simulink model "Compressor"  (R2015b)
settings: Solver=FixedStepDiscrete  StartTime=0.0  StopTime=10.0  RelTol=1e-3
undefined symbols (not defined in the file or in its folder): cp_air, etaCmax, etaCmin, gamma_air, Nc, p01, pCref, PiC, PiC_at_etaCmax, PsiMax, Q11, Q12, Q22, rComp, T01, TCref, WcCorr_at_etaCmax, WcCorrMax
settings Model: Creator=fahle  LastModifiedBy=fahle

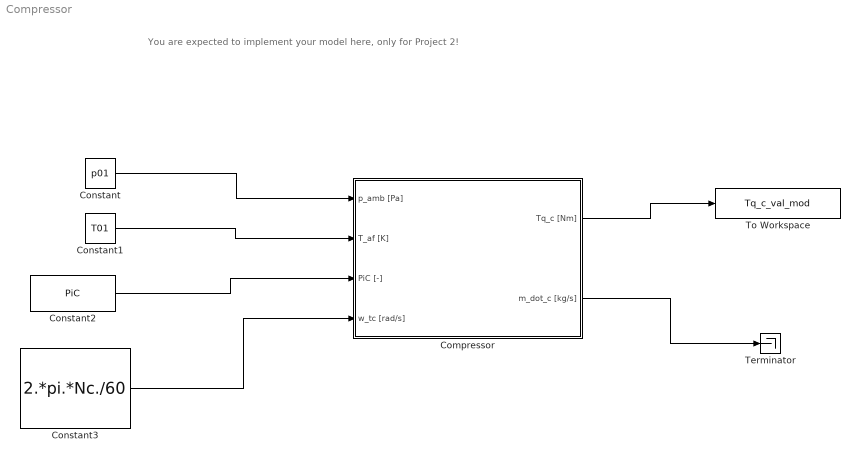
== system Compressor ==
  note: You are expected to implement your model here, only for Project 2!
  Compressor : Subsystem
  Constant : Constant  Value=p01
  Constant1 : Constant  Value=T01
  Constant2 : Constant  Value=PiC
  Constant3 : Constant  Value=2.*pi.*Nc./60
  Terminator : Terminator
  To Workspace : ToWorkspace  VariableName=Tq_c_val_mod  SampleTime=-1
      settings: Save2DSignal=2-D array (concatenate along first dimension)
  wires:
  Compressor/1(Tq_c [Nm]) -> To Workspace/1
  Compressor/2(m_dot_c [kg/s]) -> Terminator/1
  Constant3/1 -> Compressor/4(w_tc [rad/s])
  Constant2/1 -> Compressor/3(PiC [-])
  Constant1/1 -> Compressor/2(T_af [K])
  Constant/1 -> Compressor/1(p_amb [Pa])

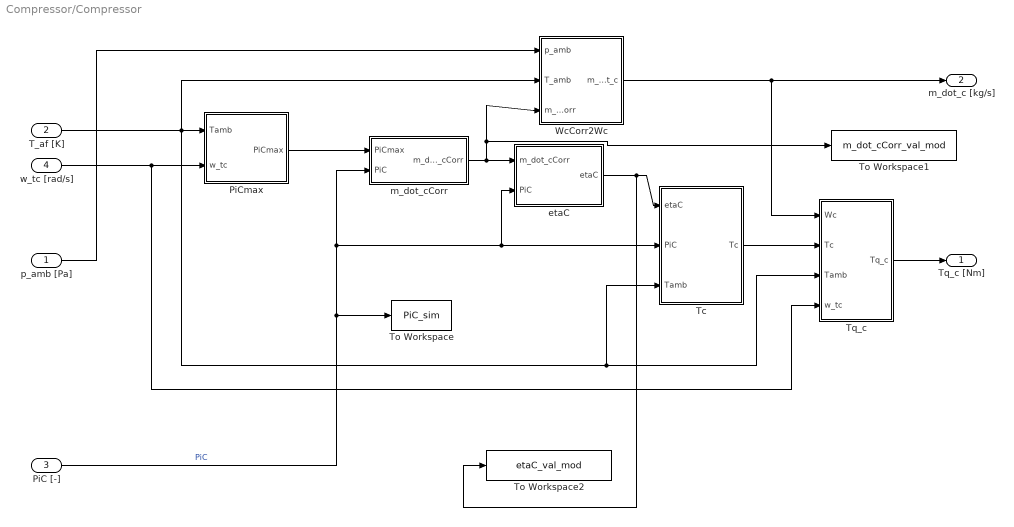
== system Compressor/Compressor ==
  p_amb [Pa] : Inport
  T_af [K] : Inport  Port=2
  PiC [-] : Inport  Port=3
  w_tc [rad/s] : Inport  Port=4
  PiCmax : Subsystem
  Tc : Subsystem
  To Workspace : ToWorkspace  VariableName=PiC_sim  SampleTime=-1
  To Workspace1 : ToWorkspace  VariableName=m_dot_cCorr_val_mod  SampleTime=-1
  To Workspace2 : ToWorkspace  VariableName=etaC_val_mod  SaveFormat=Structure With Time  SampleTime=-1
  Tq_c : Subsystem
  WcCorr2Wc : Subsystem
  etaC : Subsystem
  m_dot_cCorr : Subsystem
  Tq_c [Nm] : Outport
  m_dot_c [kg/s] : Outport  Port=2
  wires:
  T_af [K]/1 -> Tq_c/3(Tamb), Tc/3(Tamb), WcCorr2Wc/2(T_amb), PiCmax/1(Tamb)
  etaC/1(etaC) -> To Workspace2/1, Tc/1(etaC)
  p_amb [Pa]/1 -> WcCorr2Wc/1(p_amb)
  Tq_c/1(Tq_c) -> Tq_c [Nm]/1
  m_dot_cCorr/1(m_dot_cCorr) -> etaC/1(m_dot_cCorr), WcCorr2Wc/3(m_dot_cCorr), To Workspace1/1
  PiCmax/1(PiCmax) -> m_dot_cCorr/1(PiCmax)
  Tc/1(Tc) -> Tq_c/2(Tc)
  w_tc [rad/s]/1 -> Tq_c/4(w_tc), PiCmax/2(w_tc)
  PiC [-]/1 -> m_dot_cCorr/2(PiC), Tc/2(PiC), etaC/2(PiC), To Workspace/1  "PiC"
  WcCorr2Wc/1(m_dot_c) -> m_dot_c [kg/s]/1, Tq_c/1(Wc)

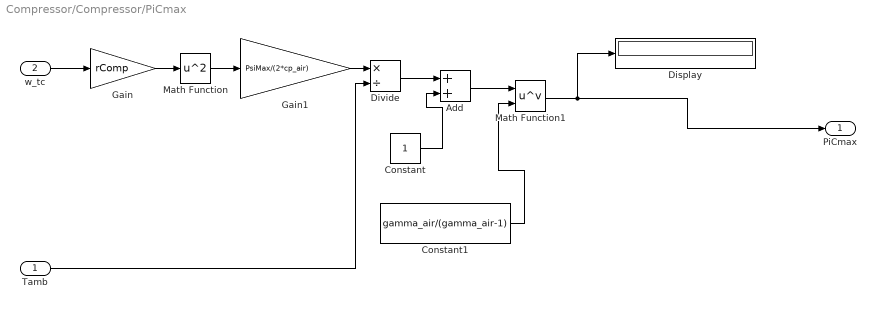
== system Compressor/Compressor/PiCmax ==
  Tamb : Inport
  w_tc : Inport  Port=2
  Add : Sum
  Constant : Constant
  Constant1 : Constant  Value=gamma_air/(gamma_air-1)
  Display : Display
  Divide : Product  Inputs=*/
  Gain : Gain  Gain=rComp
  Gain1 : Gain  Gain=PsiMax/(2*cp_air)
  Math Function : Math  Operator=square  SaturateOnIntegerOverflow=on
  Math Function1 : Math  Operator=pow  SaturateOnIntegerOverflow=on
  PiCmax : Outport
  wires:
  Math Function1/1 -> Display/1, PiCmax/1
  Tamb/1 -> Divide/2
  w_tc/1 -> Gain/1
  Gain/1 -> Math Function/1
  Math Function/1 -> Gain1/1
  Gain1/1 -> Divide/1
  Divide/1 -> Add/1
  Constant/1 -> Add/2
  Add/1 -> Math Function1/1
  Constant1/1 -> Math Function1/2

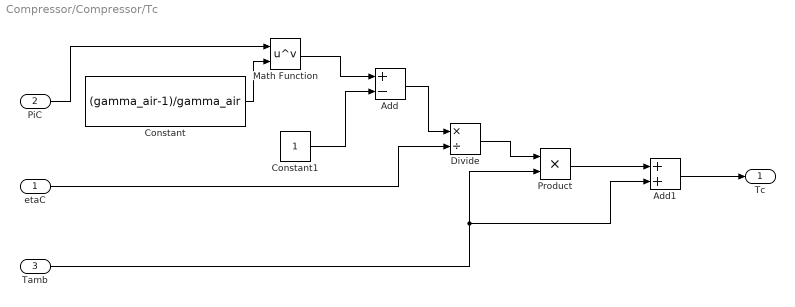
== system Compressor/Compressor/Tc ==
  etaC : Inport
  PiC : Inport  Port=2
  Tamb : Inport  Port=3
  Add : Sum  Inputs=+-
  Add1 : Sum
  Constant : Constant  Value=(gamma_air-1)/gamma_air
  Constant1 : Constant
  Divide : Product  Inputs=*/
  Math Function : Math  Operator=pow  SaturateOnIntegerOverflow=on
  Product : Product
  Tc : Outport
  wires:
  Add1/1 -> Tc/1
  PiC/1 -> Math Function/1
  etaC/1 -> Divide/2
  Tamb/1 -> Add1/2, Product/2
  Constant/1 -> Math Function/2
  Constant1/1 -> Add/2
  Math Function/1 -> Add/1
  Add/1 -> Divide/1
  Divide/1 -> Product/1
  Product/1 -> Add1/1

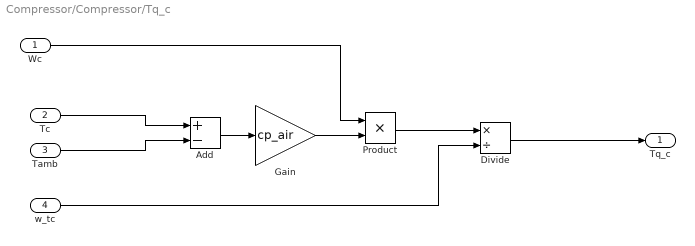
== system Compressor/Compressor/Tq_c ==
  Wc : Inport
  Tc : Inport  Port=2
  Tamb : Inport  Port=3
  w_tc : Inport  Port=4
  Add : Sum  Inputs=+-
  Divide : Product  Inputs=*/
  Gain : Gain  Gain=cp_air
  Product : Product
  Tq_c : Outport
  wires:
  w_tc/1 -> Divide/2
  Wc/1 -> Product/1
  Tc/1 -> Add/1
  Tamb/1 -> Add/2
  Add/1 -> Gain/1
  Gain/1 -> Product/2
  Product/1 -> Divide/1
  Divide/1 -> Tq_c/1

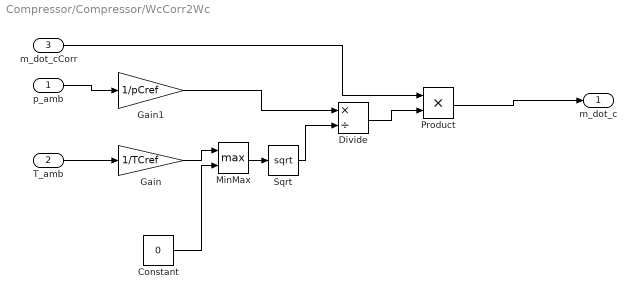
== system Compressor/Compressor/WcCorr2Wc ==
  p_amb : Inport
  T_amb : Inport  Port=2
  m_dot_cCorr : Inport  Port=3
  Constant : Constant  Value=0
  Divide : Product  Inputs=*/
  Gain : Gain  Gain=1/TCref
  Gain1 : Gain  Gain=1/pCref
  MinMax : MinMax  Function=max  Inputs=2
  Product : Product
  Sqrt : Sqrt  SaturateOnIntegerOverflow=on
  m_dot_c : Outport
  wires:
  m_dot_cCorr/1 -> Product/1
  p_amb/1 -> Gain1/1
  T_amb/1 -> Gain/1
  Product/1 -> m_dot_c/1
  Gain1/1 -> Divide/1
  Sqrt/1 -> Divide/2
  Divide/1 -> Product/2
  MinMax/1 -> Sqrt/1
  Gain/1 -> MinMax/1
  Constant/1 -> MinMax/2

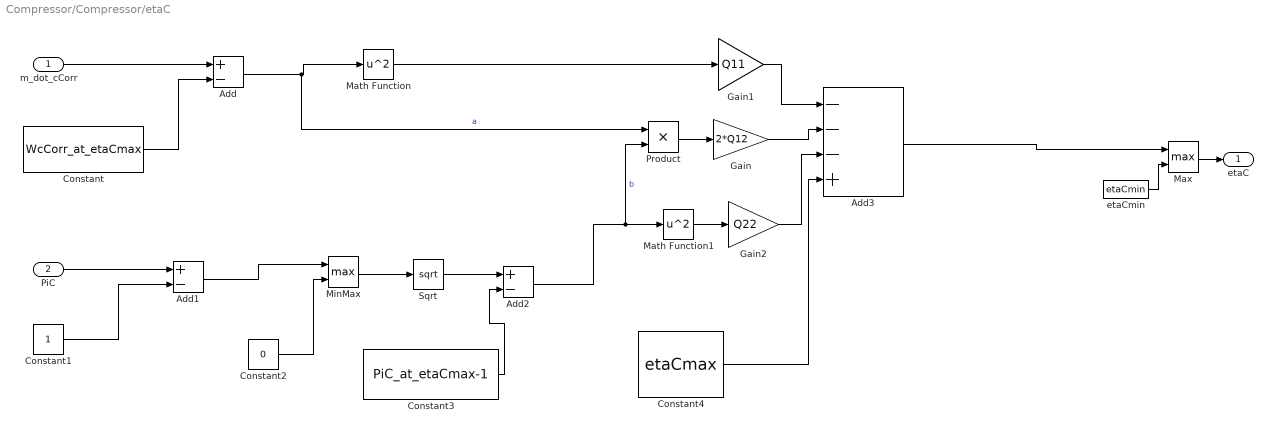
== system Compressor/Compressor/etaC ==
  m_dot_cCorr : Inport
  PiC : Inport  Port=2
  Add : Sum  Inputs=+-
  Add1 : Sum  Inputs=+-
  Add2 : Sum  Inputs=+-
  Add3 : Sum  Inputs=---+
  Constant : Constant  Value=WcCorr_at_etaCmax
  Constant1 : Constant
  Constant2 : Constant  Value=0
  Constant3 : Constant  Value=PiC_at_etaCmax-1
  Constant4 : Constant  Value=etaCmax
  Gain : Gain  Gain=2*Q12
  Gain1 : Gain  Gain=Q11
  Gain2 : Gain  Gain=Q22
  Math Function : Math  Operator=square  SaturateOnIntegerOverflow=on
  Math Function1 : Math  Operator=square  SaturateOnIntegerOverflow=on
  Max : MinMax  Function=max  Inputs=2
  MinMax : MinMax  Function=max  Inputs=2
  Product : Product
  Sqrt : Sqrt  SaturateOnIntegerOverflow=on
  etaCmin : Constant  Value=etaCmin
  etaC : Outport
  wires:
  PiC/1 -> Add1/1
  m_dot_cCorr/1 -> Add/1
  Max/1 -> etaC/1
  etaCmin/1 -> Max/2
  Add3/1 -> Max/1
  Constant/1 -> Add/2
  Add/1 -> Product/1, Math Function/1  "a"
  Constant1/1 -> Add1/2
  Constant2/1 -> MinMax/2
  Add1/1 -> MinMax/1
  MinMax/1 -> Sqrt/1
  Sqrt/1 -> Add2/1
  Constant3/1 -> Add2/2
  Math Function/1 -> Gain1/1
  Gain1/1 -> Add3/1
  Gain/1 -> Add3/2
  Gain2/1 -> Add3/3
  Add2/1 -> Product/2, Math Function1/1  "b"
  Math Function1/1 -> Gain2/1
  Product/1 -> Gain/1
  Constant4/1 -> Add3/4

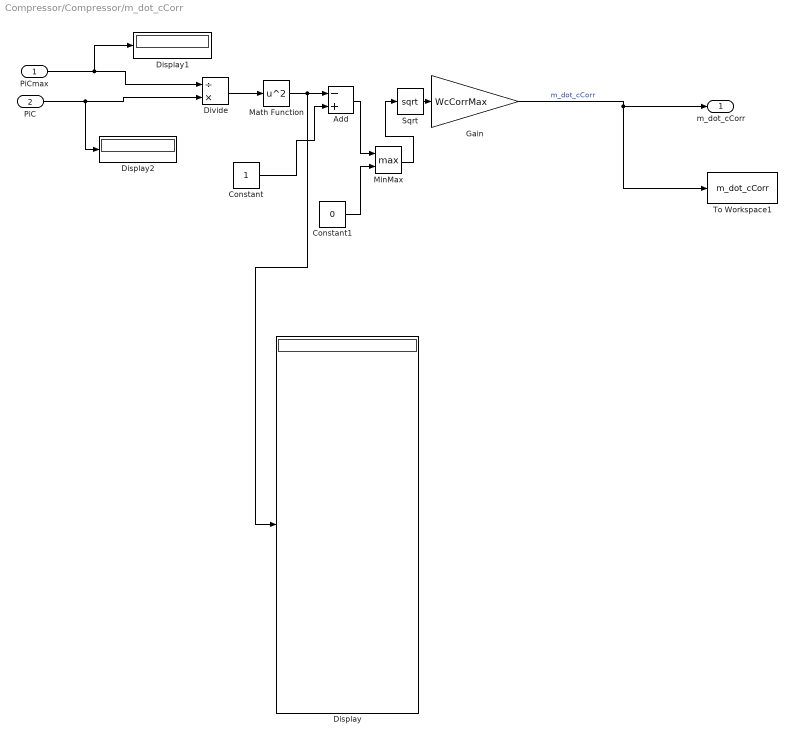
== system Compressor/Compressor/m_dot_cCorr ==
  PiCmax : Inport
  PiC : Inport  Port=2
  Add : Sum  Inputs=-+
  Constant : Constant
  Constant1 : Constant  Value=0
  Display : Display
  Display1 : Display
  Display2 : Display
  Divide : Product  Inputs=/*
  Gain : Gain  Gain=WcCorrMax
  Math Function : Math  Operator=square  SaturateOnIntegerOverflow=on
  MinMax : MinMax  Function=max  Inputs=2
  Sqrt : Sqrt  SaturateOnIntegerOverflow=on
  To Workspace1 : ToWorkspace  VariableName=m_dot_cCorr  SampleTime=-1
  m_dot_cCorr : Outport
  wires:
  PiC/1 -> Display2/1, Divide/2
  PiCmax/1 -> Display1/1, Divide/1
  Gain/1 -> m_dot_cCorr/1, To Workspace1/1  "m_dot_cCorr"
  Divide/1 -> Math Function/1
  Constant/1 -> Add/2
  Math Function/1 -> Display/1, Add/1
  Sqrt/1 -> Gain/1
  MinMax/1 -> Sqrt/1
  Add/1 -> MinMax/1
  Constant1/1 -> MinMax/2
